simulink model "PassengerCar"  (R2019b)
settings: Solver=ode1  StartTime=0  StopTime=25  FixedStep=1.0000000000000000e-003  RelTol=1e-3
InitFcn:
  | sampleTime = str2double(get_param(bdroot, 'FixedStep'));
undefined symbols (not defined in the file or in its folder): AccPedalPos, BrakePedalPos, BrakeSwitch, DiscIntNeverNeededParam, DYNA4, EngSpd, IgnitionSwitch, InitialGear, InitialSpeed, IntendedEngTrq, LeftIndicator, MainBrakePress, MaxGear, MDL, MinGear, RefAcc, RefLane, RefLatPos, RefPath, RefPathCurv, RefSpd, RefSpdPreview, RefSpdRetrospect, RightIndicator, SteeringWheelAng, SteeringWheelTrq, UserDefinedRefValue, vm_const
libraries: UtilitiesLibrary x31, simulink x18, WheelSystemModules x13, LongitudinalControllerModules x13, LateralControllerModules x7, AnimationBusselectorModules x5, EnvironmentModules x5, BasicEngineControlModules x5, MiscellaneousControlModules x5, Animation3Modules x4, AuxiliariesModules x4, TireModules x4
(part 28 of 39)

== system PassengerCar/VehicleControl/LongitudinalControl/ControlSystems/CreateOutputBus ==
  note: How to add user-defined longitudinal additional inputs to the model:
      |
      | 1. Open the block "LongitudinalControlOutput" by double-clicking on it.
      | 2. Edit the signals "UserDefined.<signalname>" inside by renaming them and setting the unit. You can also add signals to the existing ones.
      | Be careful to always use the prefix "UserDefined." for additional signals!!!
      | 3. Adjust the size of the demux-block of the user-defined signals on the left of the bus-creator so that all ports can be connected.
      | 4. Save the model to apply your changes.
  ControlOutputs : Inport
  ControlInputs : Inport  Port=2
  Phase[-] : Inport  Port=3
  UserDefinedSignals : Inport  Port=4
  Bus Selector : BusSelector  OutputSignals=AccPedalPos,BrakePedalPos,MainBrakePress,FrontLeftWheelBrakePress,FrontRightWheelBrakePress,RearLeftWheelBrakePress,RearRightWheelBrakePress,Rear2LeftWheelBrakePress,Rear2RightWheelBrakePress,Rear3LeftWheelBrakePress,Rear3RightWheelBrakePress,TrailerFrontLeftWheelBrakePress,TrailerFrontRightWheelBrakePress,TrailerRearLeftWheelBrakePress,TrailerRearRightWheelBrakePress,TrailerRear2LeftWheelBrakePress,TrailerRear2RightWheelBrakePress,TrailerRear3LeftWheelBrakePress,TrailerRear3RightWheelBrakePress,IntendedEngTrq,RefSpd,RefAcc,UserDefinedRefValue,GearRangeLowerLimit[-],GearRangeUpperLimit[-],ManualGear[-],ClutchPos[0_1],KickdownSwitch[0;1],BrakeSwitch
  Bus Selector1 : BusSelector  OutputSignals=InitialSpeed,InitialGear,ShiftingProgramSelection,InitialEngineSpd,IgnitionSwitch,Handbrake,ParkingLock,FrontDifferentialLock,RearDifferentialLock,Rear2DifferentialLock,Rear3DifferentialLock,TransferCaseLock,DayRunningLight,LowBeamLight,HighBeamLight,FogLampFront,FogLampRear,ESCSwitch,ABSSwitch,ACCSwitch,ACCRefSpd,AEBSwitch
  Demux : Demux  Outputs=2
  LongitudinalControlOutput : Subsystem  Tag=TESIS DYNAware Interface Block  mask{NeedsUpdate=off, SignalInfo=|}
      mask SignalInfo=|
      | {
      |   "Version": "4.6",
      |   "MuxedOutputBusName": "LongitudinalControl",
      |   "MuxedInputBusName": "fromCTRL",
      |   "MuxedInputSelected": false,
      |   "MuxedOutputSelected": true,
      |   "SignalData": [
      |     {
      |       "initialValue": "0.0",
      |       "name": "AccPedalPos[0_1]",
      |       "comment": "Accelerator pedal position",
      |       "minString": "",
      |       "maxString": "",
      |       "width": 1,
      |       "dataType": 0,
      |       "signalType": 0,
      |       "createSignal": false,
      |       "outputName": "AccPedalPos[0_1]",
      |       "generateSignalAccessBlock": false,
      |       "accessId": "$(parentId).$(blockName).$(outputName)"
      |     },
      |     {
      |       "initialValue": "0.0",
      |       "name": "BrakePedalPos[0_1]",
      |       "comment": "Brake pedal position",
      |       "minString": "",
      |       "maxString": "",
      |       "width": 1,
      |       "dataType": 0,
      |       "signalType": 0,
      |       "createSignal": false,
      |       "outputName": "BrakePedalPos[0_1]",
      |       "generateSignalAccessBlock": false,
      |       "accessId": "$(parentId).$(blockName).$(outputName)"
      |     },
      |     {
      |       "initialValue": "0.0",
      |       "name": "MainBrakePress[Pa]",
      |       "comment": "Main brake pressure",
      |       "minString": "",
      |       "maxString": "",
      |       "width": 1,
      |       "dataType": 0,
      |       "signalType": 0,
      |       "createSignal": false,
      |       "outputName": "MainBrakePress[Pa]",
      |       "generateSignalAccessBlock": false,
      |       "accessId": "$(parentId).$(blockName).$(outputName)"
      |     },
      |     {
      |       "initialValue": "0.0",
      |       "name": "FrontLeftWheelBrakePress[Pa]",
      |       "comment": "Front axle left wheel brake pressure",
      |       "minString": "",
      |       "maxString": "",
      |       "width": 1,
      |       "dataType": 0,
      |       "signalType": 0,
      |       "createSignal": false,
      |       "outputName": "FrontLeftWheelBrakePress[Pa]",
      |       "generateSignalAccessBlock": false,
      |       "accessId": "$(parentId).$(blockName).$(outputName)"
      |     },
      |     {
      |       "initialValue": "0.0",
      |       "name": "FrontRightWheelBrakePress[Pa]",
      |       "comment": "Front axle right wheel brake pressure",
      |       "minString": "",
      |       "maxString": "",
      |       "width": 1,
      |       "dataType": 0,
      |       "signalType": 0,
      |       "createSignal": false,
      |       "outputName": "FrontRightWheelBrakePress[Pa]",
      |       "generateSignalAccessBlock": false,
      |       "accessId": "$(parentId).$(blockName).$(outputName)"
      |     },
      |     {
      |       "initialValue": "0.0",
      |       "name": "RearLeftWheelBrakePress[Pa]",
      |       "comment": "Rear axle left wheel brake pressure",
      |       "minString": "",
      |       "maxString": "",
      |       "width": 1,
      |       "dataType": 0,
      |       "signalType": 0,
      |       "createSignal": false,
      |       "outputName": "RearLeftWheelBrakePress[Pa]",
      |       "generateSignalAccessBlock": false,
      |       "accessId": "$(parentId).$(blockName).$(outputName)"
      |     },
      |     {
      |       "initialValue": "0.0",
      |       "name": "RearRightWheelBrakePress[Pa]",
      |       "comment": "Rear axle right wheel brake pressure",
      |       "minString": "",
      |       "maxString": "",
      |       "width": 1,
      |       "dataType": 0,
      |       "signalType": 0,
      |       "createSignal": false,
      |       "outputName": "RearRightWheelBrakePress[Pa]",
      |       "generateSignalAccessBlock": false,
      |       "accessId": "$(parentId).$(blockName).$(outputName)"
      |     },
      |     {
      |       "initialValue": "0.0",
      |       "name": "Rear2LeftWheelBrakePress[Pa]",
      |       "comment": "Second rear axle left wheel brake pressure",
      |       "minString": "",
      |       "maxString": "",
      |       "width": 1,
      |       "dataType": 0,
      |       "signalType": 0,
      |       "createSignal": false,
      |       "outputName": "Rear2LeftWheelBrakePress[Pa]",
      |       "generateSignalAccessBlock": false,
      |       "accessId": "$(parentId).$(blockName).$(outputName)"
      |     },
      |     {
      |       "initialValue": "0.0",
      |       "name": "Rear2RightWheelBrakePress[Pa]",
      |       "comment": "Second rear axle right wheel brake pressure",
      |       "minString": "",
      |       "maxString": "",
      |       "width": 1,
      |       "dataType": 0,
      |       "signalType": 0,
      |       "createSignal": false,
      |       "outputName": "Rear2RightWheelBrakePress[Pa]",
      |       "generateSignalAccessBlock": false,
      |       "accessId": "$(parentId).$(blockName).$(outputName)"
      |     },
      |     {
      |       "initialValue": "0.0",
      |       "name": "Rear3LeftWheelBrakePress[Pa]",
      |       "comment": "Third rear axle left wheel brake pressure",
      |       "minString": "",
      |       "maxString": "",
      |       "width": 1,
      |       "dataType": 0,
      |       "signalType": 0,
      |       "createSignal": false,
      |       "outputName": "Rear3LeftWheelBrakePress[Pa]",
      |       "generateSignalAccessBlock": false,
      |       "accessId": "$(parentId).$(blockName).$(outputName)"
      |     },
      |     {
      |       "initialValue": "0.0",
      |       "name": "Rear3RightWheelBrakePress[Pa]",
      |       "comment": "Third rear axle right wheel brake pressure",
      |       "minString": "",
      |       "maxString": "",
      |       "width": 1,
      |       "dataType": 0,
      |       "signalType": 0,
      |       "createSignal": false,
      |       "outputName": "Rear3RightWheelBrakePress[Pa]",
      |       "generateSignalAccessBlock": false,
      |       "accessId": "$(parentId).$(blockName).$(outputName)"
      |     },
      |     {
      |       "initialValue": "0.0",
      |       "name": "TrailerFrontLeftWheelBrakePress[Pa]",
      |       "comment": "Trailer front axle left wheel brake pressure",
      |       "minString": "",
      |       "maxString": "",
      |       "width": 1,
      |       "dataType": 0,
      |       "signalType": 0,
      |       "createSignal": false,
      |       "outputName": "TrailerFrontLeftWheelBrakePress[Pa]",
      |       "generateSignalAccessBlock": false,
      |       "accessId": "$(parentId).$(blockName).$(outputName)"
      |     },
      |     {
      |       "initialValue": "0.0",
      |       "name": "TrailerFrontRightWheelBrakePress[Pa]",
      |       "comment": "Trailer front axle right wheel brake pressure",
      |       "minString": "",
      |       "maxString": "",
      |       "width": 1,
      |       "dataType": 0,
      |       "signalType": 0,
      |       "createSignal": false,
      |       "outputName": "TrailerFrontRightWheelBrakePress[Pa]",
      |       "generateSignalAccessBlock": false,
      |       "accessId": "$(parentId).$(blockName).$(outputName)"
      |     },
      |     {
      |       "initialValue": "0.0",
      |       "name": "TrailerRearLeftWheelBrakePress[Pa]",
      |       "comment": "Trailer rear axle left wheel brake pressure",
      |       "minString": "",
      |       "maxString": "",
      |       "width": 1,
      |       "dataType": 0,
      |       "signalType": 0,
      |       "createSignal": false,
      |       "outputName": "TrailerRearLeftWheelBrakePress[Pa]",
      |       "generateSignalAccessBlock": false,
      |       "accessId": "$(parentId).$(blockName).$(outputName)"
      |     },
      |     {
      |       "initialValue": "0.0",
      |       "name": "TrailerRearRightWheelBrakePress[Pa]",
      |       "comment": "Trailer rear axle right wheel brake pressure",
      |       "minString": "",
      |       "maxString": "",
      |       "width": 1,
      |       "dataType": 0,
      |       "signalType": 0,
      |       "createSignal": false,
      |       "outputName": "TrailerRearRightWheelBrakePress[Pa]",
      |       "generateSignalAccessBlock": false,
      |       "accessId": "$(parentId).$(blockName).$(outputName)"
      |     },
      |     {
      |       "initialValue": "0.0",
      |       "name": "TrailerRear2LeftWheelBrakePress[Pa]",
      |       "comment": "Trailer second rear axle left wheel brake pressure",
      |       "minString": "",
      |       "maxString": "",
      |       "width": 1,
      |       "dataType": 0,
      |       "signalType": 0,
      |       "createSignal": false,
      |       "outputName": "TrailerRear2LeftWheelBrakePress[Pa]",
      |       "generateSignalAccessBlock": false,
      |       "accessId": "$(parentId).$(blockName).$(outputName)"
      |     },
      |     {
      |       "initialValue": "0.0",
      |       "name": "TrailerRear2RightWheelBrakePress[Pa]",
      |       "comment": "Trailer second rear axle right wheel brake pressure",
      |       "minString": "",
      |       "maxString": "",
      |       "width": 1,
      |       "dataType": 0,
      |       "signalType": 0,
      |       "createSignal": false,
      |       "outputName": "TrailerRear2RightWheelBrakePress[Pa]",
      |       "generateSignalAccessBlock": false,
      |       "accessId": "$(parentId).$(blockName).$(outputName)"
      |     },
      |     {
      |       "initialValue": "0.0",
      |       "name": "TrailerRear3LeftWheelBrakePress[Pa]",
      |       "comment": "Trailer third rear axle left wheel brake pressure",
      |       "minString": "",
      |       "maxString": "",
      |       "width": 1,
      |       "dataType": 0,
      |       "signalType": 0,
      |       "createSignal": false,
      |       "outputName": "TrailerRear3LeftWheelBrakePress[Pa]",
      |       "generateSignalAccessBlock": false,
      |       "accessId": "$(parentId).$(blockName).$(outputName)"
      |     },
      |     {
      |       "initialValue": "0.0",
      |       "name": "TrailerRear3RightWheelBrakePress[Pa]",
      |       "comment": "Trailer third rear axle right wheel brake pressure",
      |       "minString": "",
      |       "maxString": "",
      |       "width": 1,
      |       "dataType": 0,
      |       "signalType": 0,
      |       "createSignal": false,
      |       "outputName": "TrailerRear3RightWheelBrakePress[Pa]",
      |       "generateSignalAccessBlock": false,
      |       "accessId": "$(parentId).$(blockName).$(outputName)"
      |     },
      |     {
      |       "initialValue": "0.0",
      |       "name": "IntendedEngTrq[Nm]",
      |       "comment": "Intended engine torque",
      |       "minString": "",
      |       "maxString": "",
      |       "width": 1,
      |       "dataType": 0,
      |       "signalType": 0,
      |       "createSignal": false,
      |       "outputName": "IntendedEngTrq[Nm]",
      |       "generateSignalAccessBlock": false,
      |       "accessId": "$(parentId).$(blockName).$(outputName)"
      |     },
      |     {
      |       "initialValue": "0.0",
      |       "name": "RefSpd[m/s]",
      |       "comment": "Vehicle reference speed",
      |       "minString": "",
      |       "maxString": "",
      |       "width": 1,
      |       "dataType": 0,
      |       "signalType": 0,
      |       "createSignal": false,
      |       "outputName": "RefSpd[m/s]",
      |       "generateSignalAccessBlock": false,
      |       "accessId": "$(parentId).$(blockName).$(outputName)"
      |     },
      |     {
      |       "initialValue": "0.0",
      |       "name": "RefAcc[m/s**2]",
      |       "comment": "",
      |       "minString": "",
      |       "maxString": "",
      |       "width": 1,
      |       "dataType": 0,
      |       "signalType": 0,
      |       "createSignal": false,
      |       "outputName": "RefAcc[m/s**2]",
      |       "generateSignalAccessBlock": false,
      |       "accessId": "$(parentId).$(blockName).$(outputName)"
      |     },
      |     {
      |       "initialValue": "0.0",
      |       "name": "UserDefinedRefValue[-]",
      |       "comment": "User-defined reference value",
      |       "minString": "",
      |       "maxString": "",
      |       "width": 1,
      |       "dataType": 0,
      |       "signalType": 0,
      |       "createSignal": false,
      |       "outputName": "UserDefinedRefValue[-]",
      |       "generateSignalAccessBlock": false,
      |       "accessId": "$(parentId).$(blockName).$(outputName)"
      |     },
      |     {
      |       "initialValue": "0.0",
      |       "name": "MinGear[-4;20]",
      |       "comment": "Minimum gear",
      |       "minString": "",
      |       "maxString": "",
      |       "width": 1,
      |       "dataType": 0,
      |       "signalType": 0,
      |       "createSignal": false,
      |       "outputName": "AutomaticGearRange.MinGear[-4;20]",
      |       "generateSignalAccessBlock": false,
      |       "accessId": "$(parentId).$(blockName).$(outputName)"
      |     },
      |     {
      |       "initialValue": "0.0",
      |       "name": "MaxGear[-4;20]",
      |       "comment": "Maximum gear",
      |       "minString": "",
      |       "maxString": "",
      |       "width": 1,
      |       "dataType": 0,
      |       "signalType": 0,
      |       "createSignal": false,
      |       "outputName": "AutomaticGearRange.MaxGear[-4;20]",
      |       "generateSignalAccessBlock": false,
      |       "accessId": "$(parentId).$(blockName).$(outputName)"
      |     },
      |     {
      |       "initialValue": "0.0",
      |       "name": "ManualGear[-4;20]",
      |       "comment": "Gear number for manual transmission",
      |       "minString": "",
      |       "maxString": "",
      |       "width": 1,
      |       "dataType": 0,
      |       "signalType": 0,
      |       "createSignal": false,
      |       "outputName": "ManualGear[-4;20]",
      |       "generateSignalAccessBlock": false,
      |       "accessId": "$(parentId).$(blockName).$(outputName)"
      |     },
      |     {
      |       "initialValue": "0.0",
      |       "name": "ClutchPos[0_1]",
      |       "comment": "Clutch position",
      |       "minString": "",
      |       "maxString": "",
      |       "width": 1,
      |       "dataType": 0,
      |       "signalType": 0,
      |       "createSignal": false,
      |       "outputName": "ClutchPos[0_1]",
      |       "generateSignalAccessBlock": false,
      |       "accessId": "$(parentId).$(blockName).$(outputName)"
      |     },
      |     {
      |       "initialValue": "0.0",
      |       "name": "KickdownSwitch[0;1]",
      |       "comment": "Kickdown switch",
      |       "minString": "",
      |       "maxString": "",
      |       "width": 1,
      |       "dataType": 0,
      |       "signalType": 0,
      |       "createSignal": false,
      |       "outputName": "KickdownSwitch[0;1]",
      |       "generateSignalAccessBlock": false,
      |       "accessId": "$(parentId).$(blockName).$(outputName)"
      |     },
      |     {
      |       "initialValue": "0.0",
      |       "name": "BrakeSwitch[1;3]",
      |       "comment": "Logical switch for brake system control, 1: Main and wheel brake pressures are calculated from the supplied brake pedal position, 2: Wheel brake pressures are calculated from the supplied main brake pressure, 3: Wheel brake pressures are supplied directly ",
      |       "minString": "",
      |       "maxString": "",
      |       "width": 1,
      |       "dataType": 0,
      |       "signalType": 0,
      |       "createSignal": false,
      |       "outputName": "BrakeSwitch[1;3]",
      |       "generateSignalAccessBlock": false,
      |       "accessId": "$(parentId).$(blockName).$(outputName)"
      |     },
      |     {
      |       "initialValue": "0.0",
      |       "name": "InitialSpeed[m/s]",
      |       "comment": "Initial vehicle speed",
      |       "minString": "",
      |       "maxString": "",
      |       "width": 1,
      |       "dataType": 0,
      |       "signalType": 0,
      |       "createSignal": false,
      |       "outputName": "InitialSpeed[m/s]",
      |       "generateSignalAccessBlock": false,
      |       "accessId": "$(parentId).$(blockName).$(outputName)"
      |     },
      |     {
      |       "initialValue": "0.0",
      |       "name": "InitialGear[-4;20]",
      |       "comment": "Initial gear",
      |       "minString": "",
      |       "maxString": "",
      |       "width": 1,
      |       "dataType": 0,
      |       "signalType": 0,
      |       "createSignal": false,
      |       "outputName": "InitialGear[-4;20]",
      |       "generateSignalAccessBlock": false,
      |       "accessId": "$(parentId).$(blockName).$(outputName)"
      |     },
      |     {
      |       "initialValue": "0.0",
      |       "name": "ShiftingProgramSelection[-]",
      |       "comment": "Selection of shifting program number",
      |       "minString": "",
      |       "maxString": "",
      |       "width": 1,
      |       "dataType": 0,
      |       "signalType": 0,
      |       "createSignal": false,
      |       "outputName": "ShiftingProgramSelection[-]",
      |       "generateSignalAccessBlock": false,
      |       "accessId": "$(parentId).$(blockName).$(outputName)"
      |     },
      |     {
      |       "initialValue": "0.0",
      |       "name": "InitialEngineSpeed[rad/s]",
      |       "comment": "Initial engine speed",
      |       "minString": "",
      |       "maxString": "",
      |       "width": 1,
      |       "dataType": 0,
      |       "signalType": 0,
      |       "createSignal": false,
      |       "outputName": "InitialEngineSpeed[rad/s]",
      |       "generateSignalAccessBlock": false,
      |       "accessId": "$(parentId).$(blockName).$(outputName)"
      |     },
      |     {
      |       "initialValue": "0.0",
      |       "name": "IgnitionSwitch[0;3]",
      |       "comment": "Ignition switch, 0: Ignition is off,  1: Only limited electric power supply, e.g for the radio, is available, 2: Normal operation mode: Full electric power supply is available, 3: Starter is activated",
      |       "minString": "",
      |       "maxString": "",
      |       "width": 1,
      |       "dataType": 0,
      |       "signalType": 0,
      |       "createSignal": false,
      |       "outputName": "IgnitionSwitch[0;3]",
      |       "generateSignalAccessBlock": false,
      |       "accessId": "$(parentId).$(blockName).$(outputName)"
      |     },
      |     {
      |       "initialValue": "0.0",
      |       "name": "Handbrake[0_1]",
      |       "comment": "Handbrake position",
      |       "minString": "",
      |       "maxString": "",
      |       "width": 1,
      |       "dataType": 0,
      |       "signalType": 0,
      |       "createSignal": false,
      |       "outputName": "Handbrake[0_1]",
      |       "generateSignalAccessBlock": false,
      |       "accessId": "$(parentId).$(blockName).$(outputName)"
      |     },
      |     {
      |       "initialValue": "0.0",
      |       "name": "ParkingLock[0;1]",
      |       "comment": "Parking lock state",
      |       "minString": "",
      |       "maxString": "",
      |       "width": 1,
      |       "dataType": 0,
      |       "signalType": 0,
      |       "createSignal": false,
      |       "outputName": "ParkingLock[0;1]",
      |       "generateSignalAccessBlock": false,
      |       "accessId": "$(parentId).$(blockName).$(outputName)"
      |     },
      |     {
      |       "initialValue": "0.0",
      |       "name": "FrontDifferentialLock[0;1]",
      |       "comment": "Front differential lock state",
      |       "minString": "",
      |       "maxString": "",
      |       "width": 1,
      |       "dataType": 0,
      |       "signalType": 0,
      |       "createSignal": false,
      |       "outputName": "FrontDifferentialLock[0;1]",
      |       "generateSignalAccessBlock": false,
      |       "accessId": "$(parentId).$(blockName).$(outputName)"
      |     },
      |     {
      |       "initialValue": "0.0",
      |       "name": "RearDifferentialLock[0;1]",
      |       "comment": "Rear differential lock state",
      |       "minString": "",
      |       "maxString": "",
      |       "width": 1,
      |       "dataType": 0,
      |       "signalType": 0,
      |       "createSignal": false,
      |       "outputName": "RearDifferentialLock[0;1]",
      |       "generateSignalAccessBlock": false,
      |       "accessId": "$(parentId).$(blockName).$(outputName)"
      |     },
      |     {
      |       "initialValue": "0.0",
      |       "name": "Rear2DifferentialLock[0;1]",
      |       "comment": "Second rear differential lock state",
      |       "minString": "",
      |       "maxString": "",
      |       "width": 1,
      |       "dataType": 0,
      |       "signalType": 0,
      |       "createSignal": false,
      |       "outputName": "Rear2DifferentialLock[0;1]",
      |       "generateSignalAccessBlock": false,
      |       "accessId": "$(parentId).$(blockName).$(outputName)"
      |     },
      |     {
      |       "initialValue": "0.0",
      |       "name": "Rear3DifferentialLock[0;1]",
      |       "comment": "Third rear differential lock state",
      |       "minString": "",
      |       "maxString": "",
      |       "width": 1,
      |       "dataType": 0,
      |       "signalType": 0,
      |       "createSignal": false,
      |       "outputName": "Rear3DifferentialLock[0;1]",
      |       "generateSignalAccessBlock": false,
      |       "accessId": "$(parentId).$(blockName).$(outputName)"
      |     },
      |     {
      |       "initialValue": "0.0",
      |       "name": "TransferCaseLock[0;1]",
      |       "comment": "Transfer case lock state",
      |       "minString": "",
      |       "maxString": "",
      |       "width": 1,
      |       "dataType": 0,
      |       "signalType": 0,
      |       "createSignal": false,
      |       "outputName": "TransferCaseLock[0;1]",
      |       "generateSignalAccessBlock": false,
      |       "accessId": "$(parentId).$(blockName).$(outputName)"
      |     },
      |     {
      |       "initialValue": "0.0",
      |       "name": "DayRunningLight[0;1]",
      |       "comment": "",
      |       "minString": "",
      |       "maxString": "",
      |       "width": 1,
      |       "dataType": 0,
      |       "signalType": 0,
      |       "createSignal": false,
      |       "outputName": "DayRunningLight[0;1]",
      |       "generateSignalAccessBlock": false,
      |       "accessId": "$(parentId).$(blockName).$(outputName)"
      |     },
      |     {
      |       "initialValue": "0.0",
      |       "name": "LowBeamLight[0;1]",
      |       "comment": "",
      |       "minString": "",
      |       "maxString": "",
      |       "width": 1,
      |       "dataType": 0,
      |       "signalType": 0,
      |       "createSignal": false,
      |       "outputName": "LowBeamLight[0;1]",
      |       "generateSignalAccessBlock": false,
      |       "accessId": "$(parentId).$(blockName).$(outputName)"
      |     },
      |     {
      |       "initialValue": "0.0",
      |       "name": "HighBeamLight[0;1]",
      |       "comment": "",
      |       "minString": "",
      |       "maxString": "",
      |       "width": 1,
      |       "dataType": 0,
      |       "signalType": 0,
      |       "createSignal": false,
      |       "outputName": "HighBeamLight[0;1]",
      |       "generateSignalAccessBlock": false,
      |       "accessId": "$(parentId).$(blockName).$(outputName)"
      |     },
      |     {
      |       "initialValue": "0.0",
      |       "name": "FogLampFront[0;1]",
      |       "comment": "",
      |       "minString": "",
      |       "maxString": "",
      |       "width": 1,
      |       "dataType": 0,
      |       "signalType": 0,
      |       "createSignal": false,
      |       "outputName": "FogLampFront[0;1]",
      |       "generateSignalAccessBlock": false,
      |       "accessId": "$(parentId).$(blockName).$(outputName)"
      |     },
      |     {
      |       "initialValue": "0.0",
      |       "name": "FogLampRear[0;1]",
      |       "comment": "",
      |       "minString": "",
      |       "maxString": "",
      |       "width": 1,
      |       "dataType": 0,
      |       "signalType": 0,
      |       "createSignal": false,
      |       "outputName": "FogLampRear[0;1]",
      |       "generateSignalAccessBlock": false,
      |       "accessId": "$(parentId).$(blockName).$(outputName)"
      |     },
      |     {
      |       "initialValue": "0.0",
      |       "name": "ESCSwitch[0;1]",
      |       "comment": "ESC activation switch",
      |       "minString": "",
      |       "maxString": "",
      |       "width": 1,
      |       "dataType": 0,
      |       "signalType": 0,
      |       "createSignal": false,
      |       "outputName": "ESCSwitch[0;1]",
      |       "generateSignalAccessBlock": false,
      |       "accessId": "$(parentId).$(blockName).$(outputName)"
      |     },
      |     {
      |       "initialValue": "0.0",
      |       "name": "ABSSwitch[0;1]",
      |       "comment": "ABS activation switch",
      |       "minString": "",
      |       "maxString": "",
      |       "width": 1,
      |       "dataType": 0,
      |       "signalType": 0,
      |       "createSignal": false,
      |       "outputName": "ABSSwitch[0;1]",
      |       "generateSignalAccessBlock": false,
      |       "accessId": "$(parentId).$(blockName).$(outputName)"
      |     },
      |     {
      |       "initialValue": "0.0",
      |       "name": "ACCSwitch[0;1]",
      |       "comment": "",
      |       "minString": "",
      |       "maxString": "",
      |       "width": 1,
      |       "dataType": 0,
      |       "signalType": 0,
      |       "createSignal": false,
      |       "outputName": "ACCSwitch[0;1]",
      |       "generateSignalAccessBlock": false,
      |       "accessId": "$(parentId).$(blockName).$(outputName)"
      |     },
      |     {
      |       "initialValue": "0.0",
      |       "name": "ACCRefSpd[m/s]",
      |       "comment": "",
      |       "minString": "",
      |       "maxString": "",
      |       "width": 1,
      |       "dataType": 0,
      |       "signalType": 0,
      |       "createSignal": false,
      |       "outputName": "ACCRefSpd[m/s]",
      |       "generateSignalAccessBlock": false,
      |       "accessId": "$(parentId).$(blockName).$(outputName)"
      |     },
      |     {
      |       "initialValue": "0.0",
      |       "name": "AEBSwitch[0;1]",
      |       "comment": "",
      |       "minString": "",
      |       "maxString": "",
      |       "width": 1,
      |       "dataType": 0,
      |       "signalType": 0,
      |       "createSignal": false,
      |       "outputName": "AEBSwitch[0;1]",
      |       "generateSignalAccessBlock": false,
      |       "accessId": "$(parentId).$(blockName).$(outputName)"
      |     },
      |     {
      |       "initialValue": "0.0",
      |       "name": "LongitudinalPhase[-]",
      |       "comment": "Longitudinal phase number",
      |       "minString": "",
      |       "maxString": "",
      |       "width": 1,
      |       "dataType": 0,
      |       "signalType": 0,
      |       "createSignal": false,
      |       "outputName": "LongitudinalPhase[-]",
      |       "generateSignalAccessBlock": false,
      |       "accessId": "$(parentId).$(blockName).$(outputName)"
      |     },
      |     {
      |       "initialValue": "0.0",
      |       "name": "UserDefined.UserDefined1[-]",
      |       "comment": "User-defined additional input 1 (can be edited by the user)",
      |       "minString": "",
      |       "maxString": "",
      |       "width": 1,
      |       "dataType": 0,
      |       "signalType": 0,
      |       "createSignal": false,
      |       "outputName": "UserDefined1[-]",
      |       "generateSignalAccessBlock": false,
      |       "accessId": "$(parentId).$(blockName).$(outputName)"
      |     },
      |     {
      |       "initialValue": "0.0",
      |       "name": "UserDefined.UserDefined2[-]",
      |       "comment": "User-defined additional input 2 (can be edited by the user)",
      |       "minString": "",
      |       "maxString": "",
      |       "width": 1,
      |       "dataType": 0,
      |       "signalType": 0,
      |       "createSignal": false,
      |       "outputName": "UserDefined2[-]",
      |       "generateSignalAccessBlock": false,
      |       "accessId": "$(parentId).$(blockName).$(outputName)"
      |     }
      |   ]
      | }
      mask prompts: NeedsUpdate "Specify, if subsystem content needs to be updated"; SignalInfo "Signal Info (json)"
      mask help: DYNA4 Interface Block Version 4.6
      mask init:
      | blockName = get_param(gcbh, 'Name');
      | parentId = DYNA4.ModelHandling.AccessID.getFromHierarchy(gcbh);
      | TD.InterfaceBlock.ModelCallbacks.GenerateContent(gcb);
      settings: DeleteFcn=TD.InterfaceBlock.ModelCallbacks.CloseGUI( gcbh );  NameChangeFcn=TD.InterfaceBlock.ModelCallbacks.BlockRenamedHandler(gcbh);  OpenFcn=TD.InterfaceBlock.ModelCallbacks.OpenGUI( gcbh );  CloseFcn=TD.InterfaceBlock.ModelCallbacks.CloseGUI( gcbh );
      mask Display:
      | image('InterfaceBlock.png','center');
      | port_label('input',1, 'AccPedalPos[0_1]');
      | port_label('input',2, 'BrakePedalPos[0_1]');
      | port_label('input',3, 'MainBrakePress[Pa]');
      | port_label('input',4, 'FrontLeftWheelBrakePress[Pa]');
      | port_label('input',5, 'FrontRightWheelBrakePress[Pa]');
      | port_label('input',6, 'RearLeftWheelBrakePress[Pa]');
      | port_label('input',7, 'RearRightWheelBrakePress[Pa]');
      | port_label('input',8, 'Rear2LeftWheelBrakePress[Pa]');
      | port_label('input',9, 'Rear2RightWheelBrakePress[Pa]');
      | port_label('input',10, 'Rear3LeftWheelBrakePress[Pa]');
      | port_label('input',11, 'Rear3RightWheelBrakePress[Pa]');
      | port_label('input',12, 'TrailerFrontLeftWheelBrakePress[Pa]');
      | port_label('input',13, 'TrailerFrontRightWheelBrakePress[Pa]');
      | port_label('input',14, 'TrailerRearLeftWheelBrakePress[Pa]');
      | port_label('input',15, 'TrailerRearRightWheelBrakePress[Pa]');
      | port_label('input',16, 'TrailerRear2LeftWheelBrakePress[Pa]');
      | port_label('input',17, 'TrailerRear2RightWheelBrakePress[Pa]');
      | port_label('input',18, 'TrailerRear3LeftWheelBrakePress[Pa]');
      | port_label('input',19, 'TrailerRear3RightWheelBrakePress[Pa]');
      | port_label('input',20, 'IntendedEngTrq[Nm]');
      | port_label('input',21, 'RefSpd[m/s]');
      | port_label('input',22, 'RefAcc[m/s**2]');
      | port_label('input',23, 'UserDefinedRefValue[-]');
      | port_label('input',24, 'MinGear[-4;20]');
      | port_label('input',25, 'MaxGear[-4;20]');
      | port_label('input',26, 'ManualGear[-4;20]');
      | port_label('input',27, 'ClutchPos[0_1]');
      | port_label('input',28, 'KickdownSwitch[0;1]');
      | port_label('input',29, 'BrakeSwitch[1;3]');
      | port_label('input',30, 'InitialSpeed[m/s]');
      | port_label('input',31, 'InitialGear[-4;20]');
      | port_label('input',32, 'ShiftingProgramSelection[-]');
      | port_label('input',33, 'InitialEngineSpeed[rad/s]');
      | port_label('input',34, 'IgnitionSwitch[0;3]');
      | port_label('input',35, 'Handbrake[0_1]');
      | port_label('input',36, 'ParkingLock[0;1]');
      | port_label('input',37, 'FrontDifferentialLock[0;1]');
      | port_label('input',38, 'RearDifferentialLock[0;1]');
      | port_label('input',39, 'Rear2DifferentialLock[0;1]');
      | port_label('input',40, 'Rear3DifferentialLock[0;1]');
      | port_label('input',41, 'TransferCaseLock[0;1]');
      | port_label('input',42, 'DayRunningLight[0;1]');
      | port_label('input',43, 'LowBeamLight[0;1]');
      | port_label('input',44, 'HighBeamLight[0;1]');
      | port_label('input',45, 'FogLampFront[0;1]');
      | port_label('input',46, 'FogLampRear[0;1]');
      | port_label('input',47, 'ESCSwitch[0;1]');
      | port_label('input',48, 'ABSSwitch[0;1]');
      | port_label('input',49, 'ACCSwitch[0;1]');
      | port_label('input',50, 'ACCRefSpd[m/s]');
      | port_label('input',51, 'AEBSwitch[0;1]');
      | port_label('input',52, 'LongitudinalPhase[-]');
      | port_label('input',53, 'UserDefined.UserDefined1[-]');
      | port_label('input',54, 'UserDefined.UserDefined2[-]');
      | port_label('output',1, 'LongitudinalControl');
  LongitudinalControl : Outport  VectorParamsAs1DForOutWhenUnconnected=off
  wires:
  Phase[-]/1 -> LongitudinalControlOutput/52(LongitudinalPhase[-]___UNIQUE_1)
  Bus Selector1/1 -> LongitudinalControlOutput/30(InitialSpeed[m/s]___UNIQUE_1)  "<InitialSpeed>"
  Bus Selector1/2 -> LongitudinalControlOutput/31(InitialGear[-4;20]___UNIQUE_1)  "<InitialGear>"
  Bus Selector1/4 -> LongitudinalControlOutput/33(InitialEngineSpeed[rad/s]___UNIQUE_1)  "<InitialEngineSpd>"
  Bus Selector1/21 -> LongitudinalControlOutput/50(ACCRefSpd[m/s]___UNIQUE_1)  "<ACCRefSpd>"
  Bus Selector1/22 -> LongitudinalControlOutput/51(AEBSwitch[0;1]___UNIQUE_1)  "<AEBSwitch>"
  ControlInputs/1 -> Bus Selector1/1
  ControlOutputs/1 -> Bus Selector/1
  LongitudinalControlOutput/1(LongitudinalControl___UNIQUE_1) -> LongitudinalControl/1
  Bus Selector/1 -> LongitudinalControlOutput/1(AccPedalPos[0_1]___UNIQUE_1)  "<AccPedalPos>"
  Bus Selector/2 -> LongitudinalControlOutput/2(BrakePedalPos[0_1]___UNIQUE_1)  "<BrakePedalPos>"
  Bus Selector/3 -> LongitudinalControlOutput/3(MainBrakePress[Pa]___UNIQUE_1)  "<MainBrakePress>"
  Bus Selector/4 -> LongitudinalControlOutput/4(FrontLeftWheelBrakePress[Pa]___UNIQUE_1)  "<FrontLeftWheelBrakePress>"
  Bus Selector/5 -> LongitudinalControlOutput/5(FrontRightWheelBrakePress[Pa]___UNIQUE_1)  "<FrontRightWheelBrakePress>"
  Bus Selector/6 -> LongitudinalControlOutput/6(RearLeftWheelBrakePress[Pa]___UNIQUE_1)  "<RearLeftWheelBrakePress>"
  Bus Selector/7 -> LongitudinalControlOutput/7(RearRightWheelBrakePress[Pa]___UNIQUE_1)  "<RearRightWheelBrakePress>"
  Bus Selector/8 -> LongitudinalControlOutput/8(Rear2LeftWheelBrakePress[Pa]___UNIQUE_1)  "<Rear2LeftWheelBrakePress>"
  Bus Selector/9 -> LongitudinalControlOutput/9(Rear2RightWheelBrakePress[Pa]___UNIQUE_1)  "<Rear2RightWheelBrakePress>"
  Bus Selector/10 -> LongitudinalControlOutput/10(Rear3LeftWheelBrakePress[Pa]___UNIQUE_1)  "<Rear3LeftWheelBrakePress>"
  Bus Selector/11 -> LongitudinalControlOutput/11(Rear3RightWheelBrakePress[Pa]___UNIQUE_1)  "<Rear3RightWheelBrakePress>"
  Bus Selector/12 -> LongitudinalControlOutput/12(TrailerFrontLeftWheelBrakePress[Pa]___UNIQUE_1)  "<TrailerFrontLeftWheelBrakePress>"
  Bus Selector/13 -> LongitudinalControlOutput/13(TrailerFrontRightWheelBrakePress[Pa]___UNIQUE_1)  "<TrailerFrontRightWheelBrakePress>"
  Bus Selector/14 -> LongitudinalControlOutput/14(TrailerRearLeftWheelBrakePress[Pa]___UNIQUE_1)  "<TrailerRearLeftWheelBrakePress>"
  Bus Selector/15 -> LongitudinalControlOutput/15(TrailerRearRightWheelBrakePress[Pa]___UNIQUE_1)  "<TrailerRearRightWheelBrakePress>"
  Bus Selector/16 -> LongitudinalControlOutput/16(TrailerRear2LeftWheelBrakePress[Pa]___UNIQUE_1)  "<TrailerRear2LeftWheelBrakePress>"
  Bus Selector/17 -> LongitudinalControlOutput/17(TrailerRear2RightWheelBrakePress[Pa]___UNIQUE_1)  "<TrailerRear2RightWheelBrakePress>"
  Bus Selector/18 -> LongitudinalControlOutput/18(TrailerRear3LeftWheelBrakePress[Pa]___UNIQUE_1)  "<TrailerRear3LeftWheelBrakePress>"
  Bus Selector/19 -> LongitudinalControlOutput/19(TrailerRear3RightWheelBrakePress[Pa]___UNIQUE_1)  "<TrailerRear3RightWheelBrakePress>"
  Bus Selector/20 -> LongitudinalControlOutput/20(IntendedEngTrq[Nm]___UNIQUE_1)  "<IntendedEngTrq>"
  Bus Selector/21 -> LongitudinalControlOutput/21(RefSpd[m/s]___UNIQUE_1)  "<RefSpd>"
  Bus Selector/22 -> LongitudinalControlOutput/22(RefAcc[m/s**2]___UNIQUE_1)  "<RefAcc>"
  Bus Selector/23 -> LongitudinalControlOutput/23(UserDefinedRefValue[-]___UNIQUE_1)  "<UserDefinedRefValue>"
  Bus Selector/24 -> LongitudinalControlOutput/24(MinGear[-4;20]___UNIQUE_1)  "<GearRangeLowerLimit[-]>"
  Bus Selector/25 -> LongitudinalControlOutput/25(MaxGear[-4;20]___UNIQUE_1)  "<GearRangeUpperLimit[-]>"
  Bus Selector/26 -> LongitudinalControlOutput/26(ManualGear[-4;20]___UNIQUE_1)  "<ManualGear[-]>"
  Bus Selector/27 -> LongitudinalControlOutput/27(ClutchPos[0_1]___UNIQUE_1)  "<ClutchPos[0_1]>"
  Bus Selector/28 -> LongitudinalControlOutput/28(KickdownSwitch[0;1]___UNIQUE_1)  "<KickdownSwitch[0;1]>"
  Bus Selector/29 -> LongitudinalControlOutput/29(BrakeSwitch[1;3]___UNIQUE_1)  "<BrakeSwitch>"
  Bus Selector1/3 -> LongitudinalControlOutput/32(ShiftingProgramSelection[-]___UNIQUE_1)  "<ShiftingProgramSelection>"
  Bus Selector1/5 -> LongitudinalControlOutput/34(IgnitionSwitch[0;3]___UNIQUE_1)  "<IgnitionSwitch>"
  Bus Selector1/6 -> LongitudinalControlOutput/35(Handbrake[0_1]___UNIQUE_1)  "<Handbrake>"
  Bus Selector1/7 -> LongitudinalControlOutput/36(ParkingLock[0;1]___UNIQUE_1)  "<ParkingLock>"
  Bus Selector1/8 -> LongitudinalControlOutput/37(FrontDifferentialLock[0;1]___UNIQUE_1)  "<FrontDifferentialLock>"
  Bus Selector1/9 -> LongitudinalControlOutput/38(RearDifferentialLock[0;1]___UNIQUE_1)  "<RearDifferentialLock>"
  Bus Selector1/10 -> LongitudinalControlOutput/39(Rear2DifferentialLock[0;1]___UNIQUE_1)  "<Rear2DifferentialLock>"
  Bus Selector1/11 -> LongitudinalControlOutput/40(Rear3DifferentialLock[0;1]___UNIQUE_1)  "<Rear3DifferentialLock>"
  Bus Selector1/12 -> LongitudinalControlOutput/41(TransferCaseLock[0;1]___UNIQUE_1)  "<TransferCaseLock>"
  Bus Selector1/18 -> LongitudinalControlOutput/47(ESCSwitch[0;1]___UNIQUE_1)  "<ESCSwitch>"
  Demux/1 -> LongitudinalControlOutput/53(UserDefined1[-]___UNIQUE_1)
  Bus Selector1/19 -> LongitudinalControlOutput/48(ABSSwitch[0;1]___UNIQUE_1)  "<ABSSwitch>"
  Bus Selector1/20 -> LongitudinalControlOutput/49(ACCSwitch[0;1]___UNIQUE_1)  "<ACCSwitch>"
  Demux/2 -> LongitudinalControlOutput/54(UserDefined2[-]___UNIQUE_1)
  UserDefinedSignals/1 -> Demux/1
  Bus Selector1/13 -> LongitudinalControlOutput/42(DayRunningLight[0;1]___UNIQUE_1)  "<DayRunningLight>"
  Bus Selector1/14 -> LongitudinalControlOutput/43(LowBeamLight[0;1]___UNIQUE_1)  "<LowBeamLight>"
  Bus Selector1/15 -> LongitudinalControlOutput/44(HighBeamLight[0;1]___UNIQUE_1)  "<HighBeamLight>"
  Bus Selector1/16 -> LongitudinalControlOutput/45(FogLampFront[0;1]___UNIQUE_1)  "<FogLampFront>"
  Bus Selector1/17 -> LongitudinalControlOutput/46(FogLampRear[0;1]___UNIQUE_1)  "<FogLampRear>"

== system PassengerCar/VehicleControl/LongitudinalControl/ControlSystems/DynaSystemInfo ==

== system PassengerCar/VehicleControl/LongitudinalControl/ControlSystems/Longitudinal Controller ==
  note: TASK_LONG_ACC_BRAKE_INPUTS = 1;
      | 	TASK_LONG_SPEED_CONTROL = 2;
      | 	TASK_LONG_ACCELERATION_CONTROL = 3;
      | 	TASK_LONG_USER_DEFINED = 4;
  "TaskIdentifiers " : Inport
  SourceIdentifiers : Inport  Port=2
  ControlInputs : Inport  Port=3
  CtrlSystemsAbscissae : Inport  Port=4
  SpeedControlParameters : Inport  Port=5
  VehicleInfoSpeedControl : Inport  Port=6
  Acceleration Brake Input : Subsystem  TreatAsAtomicUnit=on
  Acceleration Control : Subsystem  TreatAsAtomicUnit=on
  Bus Selector : BusSelector  OutputSignals=Task,Subtask
  Compute Acc Pedal Position : Subsystem
  Initialization : Subsystem  TreatAsAtomicUnit=on
  Merge : Merge  Inputs=5
  Speed Control : Subsystem  TreatAsAtomicUnit=on
  Switch Case : SwitchCase  CaseConditions={0, 1, 2, 3, 4}  ShowDefaultCase=off
  User-defined Control : Subsystem  TreatAsAtomicUnit=on
  ControlOutputs : Outport  VectorParamsAs1DForOutWhenUnconnected=off
  wires:
  User-defined Control/1(ControlOutputs) -> Merge/5
  Acceleration Control/1(ControlOutputs) -> Merge/4
  Speed Control/1(ControlOutputs) -> Merge/3
  Acceleration Brake Input/1(ControlOutputs) -> Merge/2
  Initialization/1(ControlOutputs) -> Merge/1
  SpeedControlParameters/1 -> Speed Control/2(SpeedControlParameters)
  Bus Selector/2 -> User-defined Control/4(Subtask Identifiers)  "<Subtask>"
  Bus Selector/1 -> Switch Case/1, Compute Acc Pedal Position/1(TaskIdentifier)  "<Task>"
  Switch Case/5 -> User-defined Control/Action
  Switch Case/4 -> Acceleration Control/Action
  Switch Case/3 -> Speed Control/Action
  Switch Case/1 -> Initialization/Action
  Switch Case/2 -> Acceleration Brake Input/Action
  ControlInputs/1 -> Acceleration Brake Input/1(ControlInputs), Speed Control/1(ControlInputs), Acceleration Control/1(ControlInputs), User-defined Control/1(ControlInputs)
  VehicleInfoSpeedControl/1 -> Acceleration Control/3(VehicleInfo), User-defined Control/2(VehicleInfo), Speed Control/3(VehicleInfo), Compute Acc Pedal Position/2(VehicleInfo)
  "TaskIdentifiers "/1 -> Bus Selector/1
  Compute Acc Pedal Position/1(ModifiedControlOutputs) -> ControlOutputs/1
  CtrlSystemsAbscissae/1 -> Acceleration Control/2(CtrlSystemsAbscissae)
  Merge/1 -> Compute Acc Pedal Position/3(ControlOutputs)
  SourceIdentifiers/1 -> User-defined Control/3(SourceIdentifiers)

== system PassengerCar/VehicleControl/LongitudinalControl/ControlSystemsPreprocessor/External Presetting of Controller  ==
  TaskIdentifiers : Inport
  SourceIdentifiers : Inport  Port=2
  ExtCtrlVariablesEnforced : Inport  Port=3
  Presetting Source Identifiers : Subsystem
  Presetting Task Identifiers : Subsystem
  ModifiedTaskIdentifiers : Outport  VectorParamsAs1DForOutWhenUnconnected=off
  ModifiedSourceIdentifiers : Outport  Port=2  VectorParamsAs1DForOutWhenUnconnected=off
  wires:
  Presetting Source Identifiers/1(ModifiedSourceIdentifiers) -> ModifiedSourceIdentifiers/1
  Presetting Task Identifiers/1(ModifiedTaskIdentifiers) -> ModifiedTaskIdentifiers/1
  ExtCtrlVariablesEnforced/1 -> Presetting Task Identifiers/1(ExtCtrlVariablesEnforced), Presetting Source Identifiers/1(ExtCtrlVariablesEnforced)
  TaskIdentifiers/1 -> Presetting Task Identifiers/2(TaskIdentifiers)
  SourceIdentifiers/1 -> Presetting Source Identifiers/2(SourceIdentifiers)

== system PassengerCar/VehicleControl/LongitudinalControl/ControlSystemsPreprocessor/Generation of Hold Data ==
  note: Allow InitialSpeed and InitialGear values to be used for
      | ReferenceSpeed = "Hold" and FixedGear = "Hold" modes
      | of LongitudinalManeuver parametrization.
  PhaseTrigger : Inport
  LongCTRL : Inport  Port=2
  VehicleInfo : Inport  Port=3
  ControlInputs : Inport  Port=4
  1st time step only : Memory  InitialCondition=1  InheritSampleTime=on
  Constant : Constant  Value=0
  DefaultAction Subsystem : Subsystem  TreatAsAtomicUnit=on
  Enabled Subsystem : Subsystem  TreatAsAtomicUnit=on
  InitialAction Subsystem : Subsystem  TreatAsAtomicUnit=on
  Memory : Memory  InheritSampleTime=on
  Memory1 : Memory  InheritSampleTime=on
  Merge : Merge
  Switch Case : SwitchCase
  HoldData : Outport  VectorParamsAs1DForOutWhenUnconnected=off
  wires:
  ControlInputs/1 -> InitialAction Subsystem/1(LongitudinalControlInputs)
  DefaultAction Subsystem/1(HoldLongitudinalControlInputs) -> Merge/2
  InitialAction Subsystem/1(InitialLongitudinalControlInputs) -> Merge/1
  Merge/1 -> HoldData/1
  Enabled Subsystem/1(HoldData) -> DefaultAction Subsystem/1(HoldData)
  Switch Case/2 -> DefaultAction Subsystem/Action
  Switch Case/1 -> InitialAction Subsystem/Action
  Constant/1 -> 1st time step only/1
  1st time step only/1 -> Switch Case/1
  Memory1/1 -> Enabled Subsystem/2(VehicleInfo)
  VehicleInfo/1 -> Memory1/1
  PhaseTrigger/1 -> Enabled Subsystem/Enable
  LongCTRL/1 -> Memory/1
  Memory/1 -> Enabled Subsystem/1(LongCTRL)

== system PassengerCar/VehicleControl/LongitudinalControl/ControlSystemsPreprocessor/Generation of Speed Data ==
  TaskIdentifiers : Inport
  SourceIdentifiers : Inport  Port=2
  ControlInputs : Inport  Port=3
  ReferenceSpeedParameters : Inport  Port=4
  VehicleInfo : Inport  Port=5
  TrafficInfo : Inport  Port=6
  PreviewTime[s] : Inport  Port=7
  Bus Assignment : BusAssignment  AssignedSignals=RefSpd,RefSpdPreview,RefSpdRetrospect,RefAcc,IgnitionSwitch
  Bus Selector : BusSelector  OutputSignals=RefSpd,RefSpdPreview,RefSpdRetrospect,RefAcc,IgnitionSwitch
  Demux : Demux
  Mux : Mux
  Mux1 : Mux
  ReferenceSpeedComputation : LongitudinalControllerModules/ReferenceSpeedComputation  SystemSampleTime=-1  Latency=0  AutoFrameSizeCalculation=off
  Smooth Derivative : Subsystem
  Target Speed Computation Check : Subsystem
  enforce integer values for ignition switch : Rounding  Operator=round
  isAccelerationControl : Switch  Criteria=u2 > Threshold
  isAutomatic : Switch  Criteria=u2 > Threshold
  ModifiedControlInputs : Outport  VectorParamsAs1DForOutWhenUnconnected=off
  wires:
  PreviewTime[s]/1 -> Smooth Derivative/2(PreviewTime[s])
  Target Speed Computation Check/2(isAccelerationControl) -> isAccelerationControl/2
  Bus Selector/4 -> isAccelerationControl/1  "<RefAcc>"
  Smooth Derivative/1(SmoothedRefAcc[m/s**2]) -> isAccelerationControl/3
  isAccelerationControl/1 -> Mux/4
  ReferenceSpeedComputation/2 -> Mux1/4
  ReferenceSpeedComputation/1 -> Mux1/3, Mux1/1, Mux1/2
  enforce integer values for ignition switch/1 -> Bus Assignment/6
  [IRoadInterface] -> ReferenceSpeedComputation/1
  SourceIdentifiers/1 -> Target Speed Computation Check/2(SourceIdentifiers)
  VehicleInfo/1 -> ReferenceSpeedComputation/3
  ReferenceSpeedParameters/1 -> ReferenceSpeedComputation/2
  ControlInputs/1 -> Bus Selector/1, Bus Assignment/1
  TaskIdentifiers/1 -> Target Speed Computation Check/1(TaskIdentifiers)
  Target Speed Computation Check/1(isAutomatic) -> ReferenceSpeedComputation/Enable, isAutomatic/2
  TrafficInfo/1 -> ReferenceSpeedComputation/4
  Bus Selector/1 -> Mux/1  "<RefSpd>"
  Bus Selector/2 -> Smooth Derivative/1(RefSpdPrev[m/s]), Mux/2  "<RefSpdPreview>"
  Bus Selector/3 -> Mux/3  "<RefSpdRetrospect>"
  Bus Assignment/1 -> ModifiedControlInputs/1
  Bus Selector/5 -> enforce integer values for ignition switch/1  "<IgnitionSwitch>"
  Target Speed Computation Check/3(needsSmoothedDerivative) -> Smooth Derivative/Enable
  Demux/3 -> Bus Assignment/4
  Demux/2 -> Bus Assignment/3
  Demux/4 -> Bus Assignment/5
  Demux/1 -> Bus Assignment/2
  Mux/1 -> isAutomatic/3
  Mux1/1 -> isAutomatic/1
  isAutomatic/1 -> Demux/1

== system PassengerCar/VehicleControl/LongitudinalControl/ControlSystemsPreprocessor/Switch between Data Sources ==
  note: SOURCE_NOMINALPATH = 1;
      | 	SOURCE_LANE = 2;
      | 	SOURCE_CONSTANT = 3;
      | 	SOURCE_TABLE_DISCRETE = 4;
      | 	SOURCE_TABLE_LINEAR = 5;
      | 	SOURCE_TABLE_CUBIC = 6;
      | 	SOURCE_TABLE_HAVERSINE = 7;
      | 	SOURCE_AUTOMATIC = 8;
      | 	SOURCE_SINE_TIME = 9;
      | 	SOURCE_SINE_PATH = 10;
      | 	SOURCE_HOLD = 11;
      | 	SOURCE_EXTERNAL = 12;
      | 	SOURCE_EXTERNAL_NOMINALPATH = 13;
      | 	SOURCE_EXTERNAL_LANE = 14;
  SourceIdentifiers : Inport
  ControlInputs : Inport  Port=2
  HoldData : Inport  Port=3
  ExternalData : Inport  Port=4
  Add : Sum  Inputs=3  AccumDataTypeStr=uint8
  Bus to Vector{,1..3} (4 alike) : BusToVector
  Constant : Constant
  LongitudinalControlDefaultInputs_Vector2BusObject : LongitudinalControllerModules/LongitudinalControlDefaultInputs_Vector2BusObject  SystemSampleTime=-1  Latency=0  AutoFrameSizeCalculation=off
  MinMax : MinMax  Inputs=2  OutDataTypeStr=uint8
  Multiport Switch Zero Based : MultiPortSwitch  DataPortForDefault=Additional data port  DiagnosticForDefault=None
  NonVirtualToVirtual1 : SignalConversion  ConversionOutput=Virtual bus  OverrideOpt=off
  NonVirtualToVirtual2 : SignalConversion  ConversionOutput=Virtual bus  OverrideOpt=off
  defaultValue : Constant  Value=zeros(1,vm_const('NUM_SIGNALS_LONGITUDINALMANEUVER'))
  isExternal : simulink/Logic and Bit Operations/Compare To Constant  relop=>=  const=vm_const('SOURCE_EXTERNAL')  OutDataTypeStr=uint8  ZeroCross=off
  isHold : simulink/Logic and Bit Operations/Compare To Constant  relop=>=  const=vm_const('SOURCE_HOLD')  OutDataTypeStr=uint8  ZeroCross=off
  SwitchedControlInputs : Outport  VectorParamsAs1DForOutWhenUnconnected=off
  wires:
  LongitudinalControlDefaultInputs_Vector2BusObject/1 -> SwitchedControlInputs/1
  Multiport Switch Zero Based/1 -> LongitudinalControlDefaultInputs_Vector2BusObject/1
  defaultValue/1 -> Multiport Switch Zero Based/5
  isExternal/1 -> Add/3
  isHold/1 -> Add/2
  Bus to Vector/1 -> isExternal/1, isHold/1, MinMax/2
  ControlInputs/1 -> Bus to Vector1/1
  HoldData/1 -> NonVirtualToVirtual1/1
  ExternalData/1 -> NonVirtualToVirtual2/1
  SourceIdentifiers/1 -> Bus to Vector/1
  Bus to Vector2/1 -> Multiport Switch Zero Based/3
  Bus to Vector1/1 -> Multiport Switch Zero Based/2
  MinMax/1 -> Add/1
  Constant/1 -> MinMax/1
  Bus to Vector3/1 -> Multiport Switch Zero Based/4
  NonVirtualToVirtual1/1 -> Bus to Vector2/1
  NonVirtualToVirtual2/1 -> Bus to Vector3/1
  Add/1 -> Multiport Switch Zero Based/1
